simulink model "p_controller"  (R2020a)
settings: Solver=VariableStepAuto  StartTime=0.0  StopTime=20  RelTol=1e-3
settings Model: Creator=USER  LastModifiedBy=USER

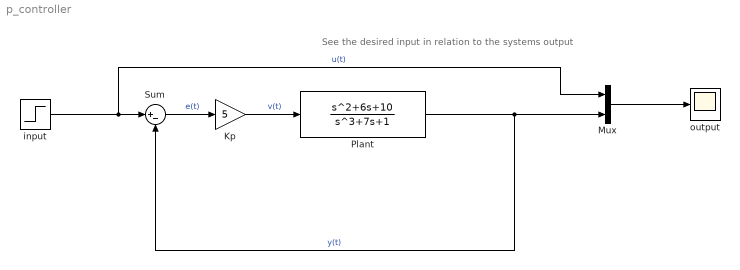
== system p_controller ==
  note: See the desired input in relation to the systems output
  Kp : Gain  Gain=5
  Mux : Mux  Inputs=2
  Plant : TransferFcn  Numerator=[1 6 10]  Denominator=[1 0 7 1]
  Sum : Sum  Inputs=|+-
  input : Step  SampleTime=0
  output : Scope
  wires:
  input/1 -> Mux/1, Sum/1  "u(t)"
  Plant/1 -> Mux/2, Sum/2  "y(t)"
  Sum/1 -> Kp/1  "e(t)"
  Kp/1 -> Plant/1  "v(t)"
  Mux/1 -> output/1
